simulink model "sim4"  (R2024a)
settings: Solver=FixedStepAuto  StartTime=0.0  StopTime=70.0  FixedStep=1e-4  RelTol=1e-3
settings Model: Creator=alexe  LastModifiedBy=alexe

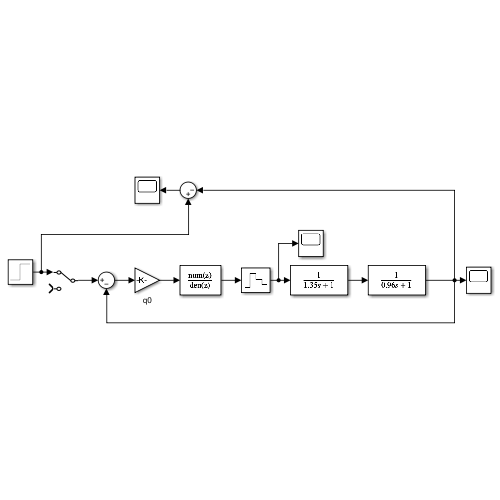
[thumbnail: Simulink's stored preview of the top-level diagram]
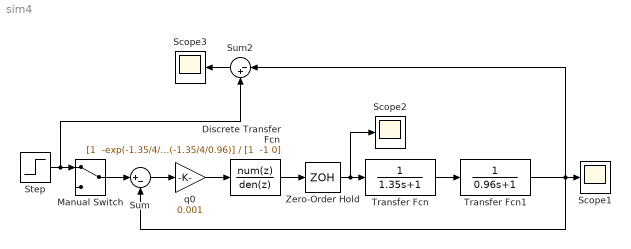
== system sim4 ==
  Discrete Transfer Fcn : DiscreteTransferFcn  Numerator="[1  -exp(-1.35/4/1.35)-exp(-1.35/4/0.96) exp(-1.35/4/1.35)*exp(-1.35/4/0.96)]"  Denominator="[1  -1 0]"
  Manual Switch : ManualSwitch
  Scope1 : Scope
  Scope2 : Scope
  Scope3 : Scope
  Step : Step  Before=1  SampleTime=0
  Sum : Sum  Inputs=|+-
  Sum2 : Sum  Inputs=|-+
  Transfer Fcn : TransferFcn  Denominator=[1.35 1]
  Transfer Fcn1 : TransferFcn  Denominator=[0.96 1]
  Zero-Order Hold : ZeroOrderHold  SampleTime=1.35/4
  q0 : Gain  Gain=0.001
  wires:
  Step/1 -> Sum2/2, Manual Switch/1
  Manual Switch/1 -> Sum/1
  q0/1 -> Discrete Transfer Fcn/1
  Discrete Transfer Fcn/1 -> Zero-Order Hold/1
  Zero-Order Hold/1 -> Scope2/1, Transfer Fcn/1
  Transfer Fcn1/1 -> Sum2/1, Sum/2, Scope1/1
  Sum/1 -> q0/1
  Sum2/1 -> Scope3/1
  Transfer Fcn/1 -> Transfer Fcn1/1
